simulink library "correlator_library"  (Simulink 6.2)
undefined symbols (not defined in the file or in its folder): BitWidthIn, BramDepth, phase_swtich_counter_width
libraries: xbsIndex_r3 x200, correlator_library x31, fft_library x11
(part 1 of 2)
settings Model: LastModifiedBy=aparsons

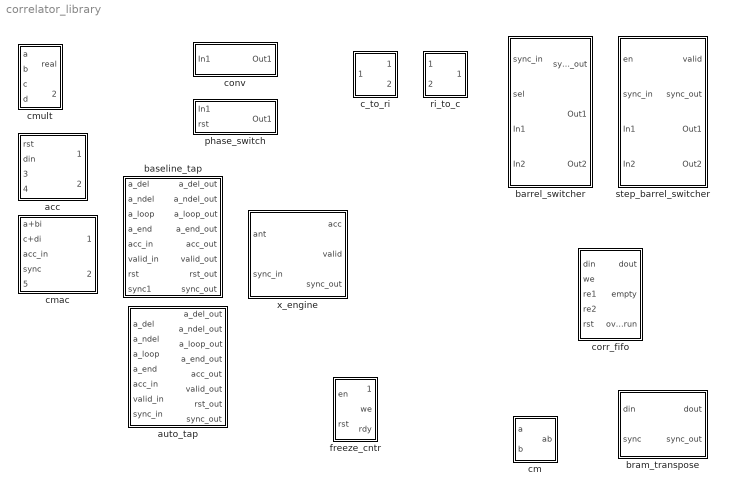
== system correlator_library ==
  acc : Subsystem  mask{BitWidthIn=18, BinPntIn=17, BitWidthOut=18, AccLen=5}
      mask prompts: BitWidthIn "Bit Width In"; BinPntIn "Binary Point In"; BitWidthOut "Bit Width Out"; AccLen "Accumulation Length"
      mask init:
      | BitGrowth = ceil(log2(AccLen));
  auto_tap : Subsystem  mask{AntNum=8, AntSep=1, BitWidthIn=18, BitWidthOut=18, AccLen=32, AddLatency=2, MultLatency=3, use_mult_core=off}
      mask prompts: AntNum "Number of Antennas"; AntSep "Antenna Seperation"; BitWidthIn "Bit Width In"; BitWidthOut "Bit Width Out"; AccLen "Accumulation Length"; AddLatency "Add Latency"; MultLatency "Mult Latency"; use_mult_core "Use Dedicated Multipliers"
      mask init:
      | BitGrowth = ceil(log2(AccLen));
      | AntBits = ceil(log2(AntNum));
      | myname = gcb;
      | set_param(myname, 'LinkStatus', 'inactive');
      | if use_mult_core
      | 	set_param([myname, '/dual_pol_cmac'], 'use_mult_core', 'on');
      | else
      | 	set_param([myname, '/dual_pol_cmac'], 'use_mult_core', 'off');
      | end
  barrel_switcher : Subsystem  mask{n_inputs=1}
      mask prompts: n_inputs "Number of Inputs:"
      mask init:
      | barrel_switcher_mask;
  baseline_tap : Subsystem  mask{AntNum=8, AntSep=1, BitWidthIn=18, BitWidthOut=18, AccLen=32, AddLatency=2, MultLatency=3, use_mult_core=off}
      mask prompts: AntNum "Number of Antennas"; AntSep "Antenna Seperation"; BitWidthIn "Bit Width In"; BitWidthOut "Bit Width Out"; AccLen "Accumulation Length"; AddLatency "Add Latency"; MultLatency "Mult Latency"; use_mult_core "Use Dedicated Multipliers"
      mask init: same as correlator_library/auto_tap
  bram_transpose : Subsystem  mask{Rows=6, Cols=2, StartCol=0}
      mask prompts: Rows "Rows of Matrix (data written in): (2^?)"; Cols "Cols of Matrix (data read out): (2^?)"; StartCol "Starting Read-out Phase (Col Number):"
  c_to_ri : Subsystem  mask{BitWidth=BitWidthIn, BinPnt=0}
      mask prompts: BitWidth "Bit Width:"; BinPnt "Binary Point:"
      mask Display:
      | port_label('input', 1, 'C')
      | port_label('output', 1, 'Re')
      | port_label('output', 2, 'Im')
  cm : Subsystem  mask{mult_latency=3, add_latency=1, use_conj=on, use_mult_core=on, n_bits=18, bin_pt=17, quantization=Round  (unbiased: +/- Inf)}
      mask prompts: mult_latency "Mult latency"; add_latency "Add latency"; use_conj "Conjugate 2nd input"; use_mult_core "Use Dedicated Multiplier"; n_bits "Sample Bitwidth"; bin_pt "Binary Point"
      mask init:
      | if use_mult_core
      | 	set_param([gcb,'/cm'], 'use_mult_core','on');
      | else
      | 	set_param([gcb,'/cm'], 'use_mult_core','off');
      | end
      | 
      | if use_conj
      | 	set_param([gcb,'/cm'],'use_conj', 'on');
      | else
      | 	set_param([gcb,'/cm'],'use_conj', 'off');
      | end
      | 
      | q = 'Round  (unbiased: +/- Inf)';
      | if quantization == 1
      |     q = 'Truncate';
      | end
      | set_param([gcb,'/cm'],'quantization', q);
      mask StyleString: edit,edit,checkbox,checkbox,edit,edit,popup(Truncate|Round  (unbiased: +/- Inf))
  cmac : Subsystem  mask{BitWidthIn=18, BitWidthOut=18, AccLen=32, MultLatency=3, AddLatency=2, use_conj=on, use_mult_core=on}
      mask prompts: BitWidthIn "Bit Width In"; BitWidthOut "Bit Width Out"; AccLen "Accumulation Length"; MultLatency "Mult Latency"; AddLatency "Add Latency"; use_conj "Conjugate 2nd Input"; use_mult_core "Use Dedicated Multipliers"
      mask init:
      | BitGrowth = ceil(log2(AccLen));
      | myname = gcb;
      | if use_conj
      | 	set_param([myname, '/cmult'], 'use_conj', 'on');
      | else
      | 	set_param([myname, '/cmult'], 'use_conj', 'off');
      | end
      | if use_mult_core
      | 	set_param([myname, '/cmult'], 'use_mult_core', 'on');
      | else
      | 	set_param([myname, '/cmult'], 'use_mult_core', 'off');
      | end
  cmult : Subsystem  mask{mult_latency=3, add_latency=1, use_conj=off, use_mult_core=on}
      mask prompts: mult_latency "Mult latency:"; add_latency "Add latency:"; use_conj "Conjugate 2nd input"; use_mult_core "Use Dedicated Multiplier"
      mask init:
      | if use_mult_core
      | 	set_param([gcb,'/ac'], 'use_embedded','on');
      | 	set_param([gcb,'/bd'], 'use_embedded','on');
      | 	set_param([gcb,'/bc'], 'use_embedded','on');
      | 	set_param([gcb,'/ad'], 'use_embedded','on');
      | else
      | 	set_param([gcb,'/ac'], 'use_embedded','off');
      | 	set_param([gcb,'/bd'], 'use_embedded','off');
      | 	set_param([gcb,'/bc'], 'use_embedded','off');
      | 	set_param([gcb,'/ad'], 'use_embedded','off');
      | end
      | 
      | if use_conj
      | 	set_param([gcb,'/real_sum'],'mode', 'Addition');
      | 	set_param([gcb,'/imag_sum'],'mode', 'Subtraction');
      | else
      | 	set_param([gcb,'/real_sum'],'mode', 'Subtraction');
      | 	set_param([gcb,'/imag_sum'],'mode', 'Addition');
      | end
  conv : Subsystem
  corr_fifo : Subsystem  mask{FIFOSize=4, percent_nbits=3}
      mask prompts: FIFOSize "Size of FIFO (2^?)"; percent_nbits "Bit Width of % Full"
      mask init:
      | if FIFOSize >= 10,
      | 	depth = [int2str(2^mod(FIFOSize, 10)), 'K'];
      | else,
      | 	depth = int2str(2^FIFOSize);
      | end
      | set_param([gcb, '/FIFO1'], 'depth', depth);
      | set_param([gcb, '/FIFO1'], 'percent_nbits', num2str(percent_nbits));
  freeze_cntr : Subsystem  mask{CounterBits=BramDepth}
      mask prompts: CounterBits "Counter Length (2^?)"
  phase_switch : Subsystem  mask{counter_width=phase_swtich_counter_width}
      mask prompts: counter_width "Counter Width:"
  ri_to_c : Subsystem  mask{test=0}
      mask prompts: test "Mask Parameter 1:"
      mask Display:
      | port_label('input', 1, 'Re')
      | port_label('input', 2, 'Im')
      | port_label('output', 1, 'C')
  step_barrel_switcher : Subsystem  mask{n_inputs=1, step_dir=Down}
      mask prompts: n_inputs "Number of Inputs: (2^?)"; step_dir "Step Direction"
      mask init:
      | step_barrel_switcher_mask;
      mask StyleString: edit,popup(Up|Down)
  x_engine : Subsystem  mask{AntNum=4, BitWidthIn=18, BitWidthOut=18, AccLen=32, AddLatency=2, MultLatency=3, use_mult_core=off}
      mask prompts: AntNum "Number of Antennas"; BitWidthIn "Bit Width of Samples In"; BitWidthOut "Bit Width of Samples Out"; AccLen "Accumulation Length"; AddLatency "Add Latency"; MultLatency "Mult Latency"; use_mult_core "Use Dedicated Multipliers"
      mask init:
      | myname = gcb;
      | set_param(myname, 'LinkStatus', 'inactive');
      | remove_all_blks(myname);
      | set_param([myname, '/ant'], 'Position', [55, 60, 85, 74]);
      | add_block('xbsIndex_r3/Constant', [myname, '/Constant'], 'Name', 'Constant');
      | set_param([myname, '/Constant'], 'Position', [15, 94, 85, 126]);
      | set_param([myname, '/Constant'], 'const', '0');
      | set_param([myname, '/Constant'], 'n_bits', '8 * BitWidthOut');
      | set_param([myname, '/Constant'], 'explicit_period', 'on');
      | add_block('xbsIndex_r3/Constant', [myname, '/Constant1'], 'Name', 'Constant1');
      | set_param([myname, '/Constant1'], 'Position', [15, 129, 85, 161]);
      | set_param([myname, '/Constant1'], 'const', '0');
      | set_param([myname, '/Constant1'], 'n_bits', '1');
      | set_param([myname, '/Constant1'], 'explicit_period', 'on');
      | set_param([myname, '/sync_in'], 'Position', [55, 185, 85, 199]);
      | x = 140;
      | for i=0:ceil(AntNum / 2)
      | 	if i == 0
      | 		stagename = 'auto_tap';
      | 	else
      | 		stagename = ['baseline_tap', num2str(i)];
      | 	end
      | 	thisblk = [myname, '/', stagename];
      | 	if i == 0
      | 		add_block('correlator_library/auto_tap', thisblk, 'Name', stagename);
      | 	else
      | 		add_block('correlator_library/baseline_tap', thisblk, 'Name', stagename);
      | 	end
      | 	set_param(thisblk, 'Position', [x, 52, x + 95, 168]);
      | 	set_param(thisblk, 'AntNum', 'AntNum');
      | 	set_param(thisblk, 'AntSep', num2str(i));
      | 	set_param(thisblk, 'BitWidthIn', 'BitWidthIn');
      | 	set_param(thisblk, 'BitWidthOut', 'BitWidthOut');
      | 	set_param(thisblk, 'AccLen', 'AccLen');
      | 	set_param(thisblk, 'AddLatency', 'AddLatency');
      | 	set_param(thisblk, 'MultLatency', 'MultLatency');
      | 	if use_mult_core,
      | 		set_param(thisblk, 'use_mult_core', 'on');
      | 	else,
      | 		set_param(thisblk, 'use_mult_core', 'off');
      | 	end
      | 	x = x + 135;
      | end
      | add_block('built-in/Terminator', [myname, '/Terminator'], 'Name', 'Terminator');
      | set_param([myname, '/Terminator'], 'Position', [x, 25, x + 20, 45]);
      | add_block('built-in/Terminator', [myname, '/Terminator1'], 'Name', 'Terminator1');
      | set_param([myname, '/Terminator1'], 'Position', [x, 65, x + 20, 85]);
      | add_block('built-in/Terminator', [myname, '/Terminator2'], 'Name', 'Terminator2');
      | set_param([myname, '/Terminator2'], 'Position', [x, 105, x + 20, 125]);
      | set_param([myname, '/acc'], 'Position', [x, 160, x + 30, 174]);
      | set_param([myname, '/valid'], 'Position', [x, 190, x + 30, 204]);
      | set_param([myname, '/sync_out'], 'Position', [x, 220, x + 30, 234]);
      | 
      | add_line(myname, 'ant/1', 'auto_tap/1', 'autorouting', 'on');
      | add_line(myname, 'ant/1', 'auto_tap/2', 'autorouting', 'on');
      | add_line(myname, 'Constant/1', 'auto_tap/5', 'autorouting', 'on');
      | add_line(myname, 'Constant1/1', 'auto_tap/6', 'autorouting', 'on');
      | add_line(myname, 'sync_in/1', 'auto_tap/7', 'autorouting', 'on');
      | add_line(myname, 'auto_tap/3', 'auto_tap/4', 'autorouting', 'on');
      | for i=1:ceil(AntNum / 2)
      | 	if i == 1
      | 		prevblk = 'auto_tap';
      | 	else
      | 		prevblk = ['baseline_tap', num2str(i-1)];
      | 	end
      | 	thisblk = ['baseline_tap', num2str(i)];
      | 	add_line(myname, [thisblk, '/3'], [prevblk, '/3'], 'autorouting', 'on');
      | 	add_line(myname, [prevblk, '/1'], [thisblk, '/1'], 'autorouting', 'on');
      | 	add_line(myname, [prevblk, '/2'], [thisblk, '/2'], 'autorouting', 'on');
      | 	add_line(myname, [prevblk, '/4'], [thisblk, '/4'], 'autorouting', 'on');
      | 	add_line(myname, [prevblk, '/5'], [thisblk, '/5'], 'autorouting', 'on');
      | 	add_line(myname, [prevblk, '/6'], [thisblk, '/6'], 'autorouting', 'on');
      | 	add_line(myname, [prevblk, '/7'], [thisblk, '/7'], 'autorouting', 'on');
      | 	add_line(myname, [prevblk, '/8'], [thisblk, '/8'], 'autorouting', 'on');
      | end
      | i = ceil(AntNum / 2);
      | thisblk = ['baseline_tap', num2str(i)];
      | add_line(myname, [thisblk, '/1'], [thisblk, '/3'], 'autorouting', 'on');
      | add_line(myname, [thisblk, '/2'], 'Terminator/1', 'autorouting', 'on');
      | add_line(myname, [thisblk, '/4'], 'Terminator1/1', 'autorouting', 'on');
      | add_line(myname, [thisblk, '/5'], 'acc/1', 'autorouting', 'on');
      | add_line(myname, [thisblk, '/6'], 'valid/1', 'autorouting', 'on');
      | add_line(myname, [thisblk, '/7'], 'Terminator2/1', 'autorouting', 'on');
      | add_line(myname, [thisblk, '/8'], 'sync_out/1', 'autorouting', 'on');

== system correlator_library/acc ==
  rst : Inport  Port=1  LatchInput=off
  din : Inport  Port=2  LatchInput=off
  acc_in : Inport  Port=3  LatchInput=off
  valid_in : Inport  Port=4  LatchInput=off
  Accumulator : xbsIndex_r3/Accumulator  n_bits=BitWidthIn + BitGrowth  overflow=Wrap  operation=Add  scale=1  explicit_period=on  period=1  rst=on  hasbypass=on  en=off  dbl_ovrd=off  show_param=off  gen_core=off  use_rpm=on
      settings: xl_area=[0, 0, 0, 0, 0, 0, 0]
  Constant : xbsIndex_r3/Constant  const=1  equ=P=C  arith_type=Unsigned  n_bits=1  bin_pt=0  opselect=C  inp2=PCIN>>17  opr=+  inp1=P  carry=CIN  iostate=0  explicit_period=on  period=1  dbl_ovrd=off
  Convert : xbsIndex_r3/Convert  arith_type="Signed  (2's comp)"  n_bits=BitWidthOut  bin_pt=BitWidthOut - BitGrowth - (BitWidthIn - BinPntIn)  quantization="Round  (unbiased: +/- Inf)"  overflow=Wrap  latency=1  explicit_period=on  period=1  dbl_ovrd=off  show_param=on  inserted_by_tool=off  pipeline=off
      settings: xl_area=[0, 0, 0, 0, 0, 0, 0]
  Convert1 : xbsIndex_r3/Convert  arith_type="Signed  (2's comp)"  n_bits=BitWidthIn + BitGrowth  bin_pt=BinPntIn  quantization="Round  (unbiased: +/- Inf)"  overflow=Wrap  latency=1  explicit_period=off  period=1  dbl_ovrd=off  show_param=on  inserted_by_tool=off  pipeline=off
      settings: xl_area=[0, 0, 0, 0, 0, 0, 0]
  Delay : xbsIndex_r3/Delay  Orientation=up  latency=1  reg_retiming=off  explicit_period=off  period=1  en=off  accept_only_valid=off  init_zero=on  dbl_ovrd=off  show_param=off
      settings: xl_area=[0, 0, 0, 0, 0, 0, 0]
  Delay1 : xbsIndex_r3/Delay  latency=1  reg_retiming=off  explicit_period=off  period=1  en=off  accept_only_valid=off  init_zero=on  dbl_ovrd=off  show_param=off
      settings: xl_area=[0, 0, 0, 0, 0, 0, 0]
  Mux2 : xbsIndex_r3/Mux  inputs=2  precision=Full  arith_type="Signed  (2's comp)"  n_bits=0  bin_pt=0  quantization="Round  (unbiased: +/- Inf)"  overflow=Wrap  latency=2  explicit_period=on  period=1  en=off  dbl_ovrd=off  show_param=off  mux_type=off  use_rpm=off  gen_core=off
      settings: xl_area=[0, 0, 0, 0, 0, 0, 0]
  Mux3 : xbsIndex_r3/Mux  inputs=2  precision=Full  arith_type="Signed  (2's comp)"  n_bits=0  bin_pt=0  quantization=Truncate  overflow=Wrap  latency=2  explicit_period=on  period=1  en=off  dbl_ovrd=off  show_param=off  mux_type=off  use_rpm=off  gen_core=off
      settings: xl_area=[0, 0, 0, 0, 0, 0, 0]
  acc_out : Outport
  valid_out : Outport  Port=2
  wires:
  Accumulator/1 -> Convert/1
  Mux2/1 -> acc_out/1
  acc_in/1 -> Mux2/2
  valid_in/1 -> Mux3/2
  Constant/1 -> Mux3/3
  Mux3/1 -> valid_out/1
  din/1 -> Convert1/1
  rst/1 -> Delay1/1
  Delay/1 -> Mux3/1, Mux2/1
  Convert/1 -> Mux2/3
  Convert1/1 -> Accumulator/1
  Delay1/1 -> Accumulator/2, Delay/1

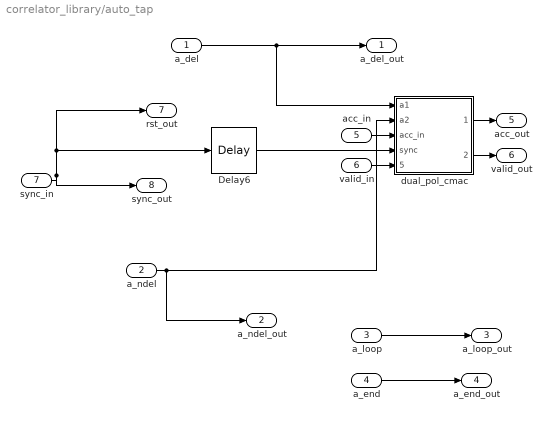
== system correlator_library/auto_tap ==
  a_del : Inport  Port=1  LatchInput=off
  a_ndel : Inport  Port=2  LatchInput=off
  a_loop : Inport  Port=3  LatchInput=off
  a_end : Inport  Port=4  LatchInput=off
  acc_in : Inport  Port=5  LatchInput=off
  valid_in : Inport  Port=6  LatchInput=off
  sync_in : Inport  Port=7  LatchInput=off
  Delay6 : xbsIndex_r3/Delay  latency=1  reg_retiming=off  explicit_period=off  period=1  en=off  accept_only_valid=off  init_zero=on  dbl_ovrd=off  show_param=off
      settings: xl_area=[0, 0, 0, 0, 0, 0, 0]
  dual_pol_cmac : Subsystem  mask{BitWidthIn=BitWidthIn, BitWidthOut=BitWidthOut, AccLen=AccLen, MultLatency=MultLatency, AddLatency=AddLatency, use_mult_core=off}
      mask prompts: BitWidthIn "Bit Width of Sample In"; BitWidthOut "Bit Width of Sample Out"; AccLen "Accumulation Length"; MultLatency "Mult Latency"; AddLatency "Add Latency"; use_mult_core "Use Dedicated Multipliers"
      mask init:
      | myname = gcb;
      | for i=1:4
      | 	if i == 1
      | 		thisblk = '/cmac';
      | 	elseif i == 2
      | 		thisblk = '/cmac1';
      | 	elseif i == 3
      | 		thisblk = '/cmac2';
      | 	elseif i == 4
      | 		thisblk = '/cmac3';
      | 	end
      | 	if use_mult_core
      | 		set_param([myname, thisblk], 'use_mult_core', 'on');
      | 	else
      | 		set_param([myname, thisblk], 'use_mult_core', 'off');
      | 	end
      | end
  a_del_out : Outport
  a_ndel_out : Outport  Port=2
  a_loop_out : Outport  Port=3
  a_end_out : Outport  Port=4
  acc_out : Outport  Port=5
  valid_out : Outport  Port=6
  rst_out : Outport  Port=7
  sync_out : Outport  Port=8
  wires:
  a_loop/1 -> a_loop_out/1
  a_end/1 -> a_end_out/1
  a_ndel/1 -> a_ndel_out/1, dual_pol_cmac/2(a2)
  valid_in/1 -> dual_pol_cmac/5(valid_in)
  dual_pol_cmac/2(valid_out) -> valid_out/1
  acc_in/1 -> dual_pol_cmac/3(acc_in)
  dual_pol_cmac/1(acc_out) -> acc_out/1
  a_del/1 -> a_del_out/1, dual_pol_cmac/1(a1)
  sync_in/1 -> rst_out/1, Delay6/1, sync_out/1
  Delay6/1 -> dual_pol_cmac/4(sync)

== system correlator_library/barrel_switcher ==
  sync_in : Inport  Port=1  LatchInput=off
  sel : Inport  Port=2  LatchInput=off
  In1 : Inport  Port=3  LatchInput=off
  In2 : Inport  Port=4  LatchInput=off
  Delay_sync : xbsIndex_r3/Delay  latency=1  reg_retiming=off  explicit_period=off  period=1  en=off  accept_only_valid=off  init_zero=on  dbl_ovrd=off  show_param=off
      settings: xl_area=[0, 0, 0, 0, 0, 0, 0]
  Mux11 : xbsIndex_r3/Mux  inputs=2  precision=Full  arith_type="Signed  (2's comp)"  n_bits=8  bin_pt=2  quantization=Truncate  overflow=Wrap  latency=1  explicit_period=off  period=1  en=off  dbl_ovrd=off  show_param=off  mux_type=off  use_rpm=off  gen_core=off
      settings: xl_area=[0, 0, 0, 0, 0, 0, 0]
  Mux21 : xbsIndex_r3/Mux  inputs=2  precision=Full  arith_type="Signed  (2's comp)"  n_bits=8  bin_pt=2  quantization=Truncate  overflow=Wrap  latency=1  explicit_period=off  period=1  en=off  dbl_ovrd=off  show_param=off  mux_type=off  use_rpm=off  gen_core=off
      settings: xl_area=[0, 0, 0, 0, 0, 0, 0]
  Slice1 : xbsIndex_r3/Slice  mode=Upper Bit Location + Width  nbits=1  bit1=-0  base1=MSB of Input  bit0=0  base0=LSB of Input  boolean_output=off  explicit_period=off  period=1  dbl_ovrd=off
  sync_out : Outport
  Out1 : Outport  Port=2
  Out2 : Outport  Port=3
  wires:
  sync_in/1 -> Delay_sync/1
  Delay_sync/1 -> sync_out/1
  sel/1 -> Slice1/1
  Slice1/1 -> Mux11/1, Mux21/1
  In1/1 -> Mux11/2, Mux21/3
  Mux11/1 -> Out1/1
  In2/1 -> Mux21/2, Mux11/3
  Mux21/1 -> Out2/1

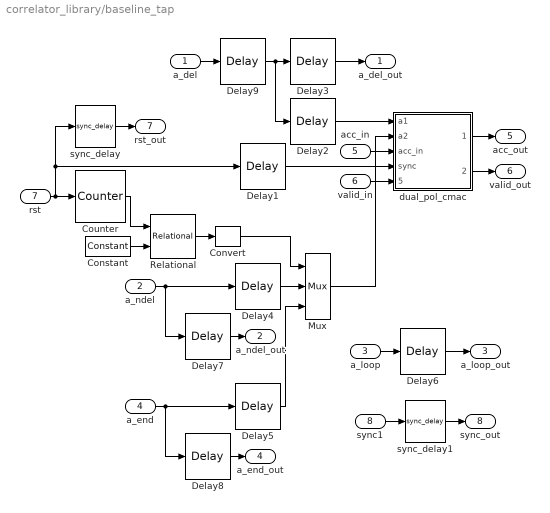
== system correlator_library/baseline_tap ==
  a_del : Inport  Port=1  LatchInput=off
  a_ndel : Inport  Port=2  LatchInput=off
  a_loop : Inport  Port=3  LatchInput=off
  a_end : Inport  Port=4  LatchInput=off
  acc_in : Inport  Port=5  LatchInput=off
  valid_in : Inport  Port=6  LatchInput=off
  rst : Inport  Port=7  LatchInput=off
  sync1 : Inport  Port=8  LatchInput=off
  Constant : xbsIndex_r3/Constant  const=(AntNum - AntSep) * AccLen  equ=P=C  arith_type=Unsigned  n_bits=AntBits + BitGrowth  bin_pt=0  opselect=C  inp2=PCIN>>17  opr=+  inp1=P  carry=CIN  iostate=0  explicit_period=off  period=1  dbl_ovrd=off
  Convert : xbsIndex_r3/Convert  arith_type=Unsigned  n_bits=1  bin_pt=0  quantization=Truncate  overflow=Wrap  latency=0  explicit_period=off  period=1  dbl_ovrd=off  show_param=off  inserted_by_tool=off  pipeline=off
      settings: xl_area=[0, 0, 0, 0, 0, 0, 0]
  Counter : xbsIndex_r3/Counter  cnt_type=Count Limited  n_bits=AntBits + BitGrowth  bin_pt=0  arith_type=Unsigned  start_count=0  cnt_to=AntNum * AccLen - 1  cnt_by_val=1  operation=Up  explicit_period=off  period=1  load_pin=off  rst=on  en=off  dbl_ovrd=off  show_param=off  use_rpm=on  gen_core=off
      settings: xl_area=[0, 0, 0, 0, 0, 0, 0]
  Delay1 : xbsIndex_r3/Delay  latency=2  reg_retiming=off  explicit_period=off  period=1  en=off  accept_only_valid=off  init_zero=on  dbl_ovrd=off  show_param=off
      settings: xl_area=[0, 0, 0, 0, 0, 0, 0]
  Delay2 : xbsIndex_r3/Delay  latency=2  reg_retiming=off  explicit_period=off  period=1  en=off  accept_only_valid=off  init_zero=on  dbl_ovrd=off  show_param=off
      settings: xl_area=[0, 0, 0, 0, 0, 0, 0]
  Delay3 : xbsIndex_r3/Delay  latency=1  reg_retiming=off  explicit_period=off  period=1  en=off  accept_only_valid=off  init_zero=on  dbl_ovrd=off  show_param=off
      settings: xl_area=[0, 0, 0, 0, 0, 0, 0]
  Delay{4..5,7..8} (4 alike) : xbsIndex_r3/Delay  latency=1  reg_retiming=off  explicit_period=on  period=1  en=off  accept_only_valid=off  init_zero=on  dbl_ovrd=off  show_param=off
      settings: xl_area=[0, 0, 0, 0, 0, 0, 0]
  Delay6 : xbsIndex_r3/Delay  latency=2 * AccLen  reg_retiming=off  explicit_period=off  period=1  en=off  accept_only_valid=off  init_zero=on  dbl_ovrd=off  show_param=off
      settings: xl_area=[0, 0, 0, 0, 0, 0, 0]
  Delay9 : xbsIndex_r3/Delay  latency=2 * AccLen  reg_retiming=off  explicit_period=off  period=1  en=off  accept_only_valid=off  init_zero=on  dbl_ovrd=off  show_param=off
      settings: xl_area=[0, 0, 0, 0, 0, 0, 0]
  Mux : xbsIndex_r3/Mux  inputs=2  precision=Full  arith_type="Signed  (2's comp)"  n_bits=8  bin_pt=2  quantization=Truncate  overflow=Wrap  latency=1  explicit_period=off  period=1  en=off  dbl_ovrd=off  show_param=off  mux_type=off  use_rpm=off  gen_core=off
      settings: xl_area=[0, 0, 0, 0, 0, 0, 0]
  Relational : xbsIndex_r3/Relational  mode=a>=b  latency=1  explicit_period=off  period=1  en=off  dbl_ovrd=off  show_param=off
      settings: xl_area=[0, 0, 0, 0, 0, 0, 0]
  dual_pol_cmac : Subsystem  mask{BitWidthIn=BitWidthIn, BitWidthOut=BitWidthOut, AccLen=AccLen, MultLatency=MultLatency, AddLatency=AddLatency, use_mult_core=off}
      mask prompts: BitWidthIn "Bit Width of Sample In"; BitWidthOut "Bit Width of Sample Out"; AccLen "Accumulation Length"; MultLatency "Mult Latency"; AddLatency "Add Latency"; use_mult_core "Use Dedicated Multipliers"
      mask init: same as correlator_library/auto_tap/dual_pol_cmac
  sync_delay : fft_library/sync_delay  DelayLen=AccLen + 1
  sync_delay1 : fft_library/sync_delay  DelayLen=2 * AccLen
  a_del_out : Outport
  a_ndel_out : Outport  Port=2
  a_loop_out : Outport  Port=3
  a_end_out : Outport  Port=4
  acc_out : Outport  Port=5
  valid_out : Outport  Port=6
  rst_out : Outport  Port=7
  sync_out : Outport  Port=8
  wires:
  Delay4/1 -> Mux/2
  Delay5/1 -> Mux/3
  Delay9/1 -> Delay2/1, Delay3/1
  Delay2/1 -> dual_pol_cmac/1(a1)
  Mux/1 -> dual_pol_cmac/2(a2)
  Counter/1 -> Relational/1
  Constant/1 -> Relational/2
  Relational/1 -> Convert/1
  Convert/1 -> Mux/1
  Delay1/1 -> dual_pol_cmac/4(sync)
  rst/1 -> Counter/1, Delay1/1, sync_delay/1
  a_del/1 -> Delay9/1
  dual_pol_cmac/1(acc_out) -> acc_out/1
  acc_in/1 -> dual_pol_cmac/3(acc_in)
  dual_pol_cmac/2(valid_out) -> valid_out/1
  valid_in/1 -> dual_pol_cmac/5(valid_in)
  a_ndel/1 -> Delay4/1, Delay7/1
  a_end/1 -> Delay5/1, Delay8/1
  a_loop/1 -> Delay6/1
  Delay6/1 -> a_loop_out/1
  Delay3/1 -> a_del_out/1
  Delay7/1 -> a_ndel_out/1
  Delay8/1 -> a_end_out/1
  sync_delay/1 -> rst_out/1
  sync_delay1/1 -> sync_out/1
  sync1/1 -> sync_delay1/1

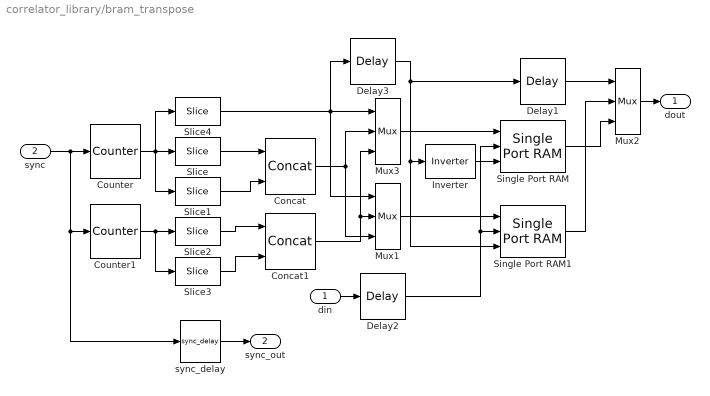
== system correlator_library/bram_transpose ==
  din : Inport  Port=1  LatchInput=off
  sync : Inport  Port=2  LatchInput=off
  Concat : xbsIndex_r3/Concat  num_inputs=2  explicit_period=off  period=1  dbl_ovrd=off
  Concat1 : xbsIndex_r3/Concat  num_inputs=2  explicit_period=off  period=1  dbl_ovrd=off
  Counter : xbsIndex_r3/Counter  cnt_type=Free Running  n_bits=Rows + Cols + 1  bin_pt=0  arith_type=Unsigned  start_count=0  cnt_to=Inf  cnt_by_val=1  operation=Up  explicit_period=on  period=1  load_pin=off  rst=on  en=off  dbl_ovrd=off  show_param=off  use_rpm=on  gen_core=off
      settings: xl_area=[0, 0, 0, 0, 0, 0, 0]
  Counter1 : xbsIndex_r3/Counter  cnt_type=Free Running  n_bits=Rows + Cols + 1  bin_pt=0  arith_type=Unsigned  start_count=StartCol  cnt_to=Inf  cnt_by_val=1  operation=Up  explicit_period=on  period=1  load_pin=off  rst=on  en=off  dbl_ovrd=off  show_param=on  use_rpm=on  gen_core=off
      settings: xl_area=[0, 0, 0, 0, 0, 0, 0]
  Delay1 : xbsIndex_r3/Delay  latency=3  reg_retiming=off  explicit_period=off  period=1  en=off  accept_only_valid=off  init_zero=on  dbl_ovrd=off  show_param=off
      settings: xl_area=[0, 0, 0, 0, 0, 0, 0]
  Delay2 : xbsIndex_r3/Delay  latency=1  reg_retiming=off  explicit_period=off  period=1  en=off  accept_only_valid=off  init_zero=on  dbl_ovrd=off  show_param=off
      settings: xl_area=[0, 0, 0, 0, 0, 0, 0]
  Delay3 : xbsIndex_r3/Delay  latency=1  reg_retiming=off  explicit_period=off  period=1  en=off  accept_only_valid=off  init_zero=on  dbl_ovrd=off  show_param=off
      settings: xl_area=[0, 0, 0, 0, 0, 0, 0]
  Inverter : xbsIndex_r3/Inverter  latency=0  explicit_period=off  period=1  en=off  dbl_ovrd=off  show_param=off
      settings: xl_area=[0, 0, 0, 0, 0, 0, 0]
  Mux1 : xbsIndex_r3/Mux  inputs=2  precision=Full  arith_type="Signed  (2's comp)"  n_bits=8  bin_pt=2  quantization=Truncate  overflow=Wrap  latency=1  explicit_period=off  period=1  en=off  dbl_ovrd=off  show_param=off  mux_type=off  use_rpm=off  gen_core=off
      settings: xl_area=[0, 0, 0, 0, 0, 0, 0]
  Mux2 : xbsIndex_r3/Mux  inputs=2  precision=Full  arith_type="Signed  (2's comp)"  n_bits=8  bin_pt=2  quantization=Truncate  overflow=Wrap  latency=1  explicit_period=off  period=1  en=off  dbl_ovrd=off  show_param=off  mux_type=off  use_rpm=off  gen_core=off
      settings: xl_area=[0, 0, 0, 0, 0, 0, 0]
  Mux3 : xbsIndex_r3/Mux  inputs=2  precision=Full  arith_type="Signed  (2's comp)"  n_bits=8  bin_pt=2  quantization=Truncate  overflow=Wrap  latency=1  explicit_period=off  period=1  en=off  dbl_ovrd=off  show_param=off  mux_type=off  use_rpm=off  gen_core=off
      settings: xl_area=[0, 0, 0, 0, 0, 0, 0]
  Single Port RAM : xbsIndex_r3/Single Port RAM  depth=2^(Rows + Cols)  initVector=0  write_mode=Read Before Write  latency=3  init_zero=on  explicit_period=off  period=1  rst=off  init_reg=0  en=off  dbl_ovrd=off  show_param=off  distributed_mem=off  use_rpm=off  gen_core=off
      settings: xl_area=[0, 0, 0, 0, 0, 0, 0]
  Single Port RAM1 : xbsIndex_r3/Single Port RAM  depth=2^(Rows + Cols)  initVector=0  write_mode=Read Before Write  latency=3  init_zero=on  explicit_period=off  period=1  rst=off  init_reg=0  en=off  dbl_ovrd=off  show_param=off  distributed_mem=off  use_rpm=off  gen_core=off
      settings: xl_area=[0, 0, 0, 0, 0, 0, 0]
  Slice : xbsIndex_r3/Slice  mode=Upper Bit Location + Width  nbits=Cols  bit1=-1  base1=MSB of Input  bit0=0  base0=LSB of Input  boolean_output=off  explicit_period=off  period=1  dbl_ovrd=off
  Slice1 : xbsIndex_r3/Slice  mode=Lower Bit Location + Width  nbits=Rows  bit1=0  base1=MSB of Input  bit0=0  base0=LSB of Input  boolean_output=off  explicit_period=off  period=1  dbl_ovrd=off
  Slice2 : xbsIndex_r3/Slice  mode=Lower Bit Location + Width  nbits=Cols  bit1=-1  base1=MSB of Input  bit0=0  base0=LSB of Input  boolean_output=off  explicit_period=off  period=1  dbl_ovrd=off
  Slice3 : xbsIndex_r3/Slice  mode=Upper Bit Location + Width  nbits=Rows  bit1=-1  base1=MSB of Input  bit0=0  base0=LSB of Input  boolean_output=off  explicit_period=off  period=1  dbl_ovrd=off
  Slice4 : xbsIndex_r3/Slice  mode=Upper Bit Location + Width  nbits=1  bit1=0  base1=MSB of Input  bit0=0  base0=LSB of Input  boolean_output=on  explicit_period=off  period=1  dbl_ovrd=off
  sync_delay : fft_library/sync_delay  DelayLen=2^(Rows + Cols) + 5
  dout : Outport
  sync_out : Outport  Port=2
  wires:
  Slice3/1 -> Concat1/2
  Slice2/1 -> Concat1/1
  Inverter/1 -> Single Port RAM/3
  Mux2/1 -> dout/1
  Delay1/1 -> Mux2/1
  din/1 -> Delay2/1
  Single Port RAM/1 -> Mux2/3
  Single Port RAM1/1 -> Mux2/2
  Mux1/1 -> Single Port RAM1/1
  Mux3/1 -> Single Port RAM/1
  sync/1 -> Counter/1, Counter1/1, sync_delay/1
  Slice1/1 -> Concat/2
  Slice/1 -> Concat/1
  Concat1/1 -> Mux1/2, Mux3/3
  Concat/1 -> Mux1/3, Mux3/2
  Slice4/1 -> Mux1/1, Mux3/1, Delay3/1
  Delay2/1 -> Single Port RAM/2, Single Port RAM1/2
  Delay3/1 -> Single Port RAM1/3, Inverter/1, Delay1/1
  Counter/1 -> Slice/1, Slice4/1, Slice1/1
  Counter1/1 -> Slice2/1, Slice3/1
  sync_delay/1 -> sync_out/1

== system correlator_library/c_to_ri ==
  In1 : Inport  Port=1  LatchInput=off
  Reinterpret : xbsIndex_r3/Reinterpret  force_arith_type=on  arith_type="Signed  (2's comp)"  force_bin_pt=on  bin_pt=BinPnt  force_valid=on
  Reinterpret1 : xbsIndex_r3/Reinterpret  force_arith_type=on  arith_type="Signed  (2's comp)"  force_bin_pt=on  bin_pt=BinPnt  force_valid=on
  Slice : xbsIndex_r3/Slice  mode=Upper Bit Location + Width  nbits=BitWidth  bit1=0  base1=MSB of Input  bit0=0  base0=LSB of Input  boolean_output=off  explicit_period=off  period=1  dbl_ovrd=off
  Slice1 : xbsIndex_r3/Slice  mode=Lower Bit Location + Width  nbits=BitWidth  bit1=0  base1=MSB of Input  bit0=0  base0=LSB of Input  boolean_output=off  explicit_period=off  period=1  dbl_ovrd=off
  Out1 : Outport
  Out2 : Outport  Port=2
  wires:
  In1/1 -> Slice1/1, Slice/1
  Reinterpret1/1 -> Out2/1
  Reinterpret/1 -> Out1/1
  Slice1/1 -> Reinterpret1/1
  Slice/1 -> Reinterpret/1

== system correlator_library/cm ==
  a : Inport  Port=1  LatchInput=off
  b : Inport  Port=2  LatchInput=off
  c_to_ri : correlator_library/c_to_ri  BitWidth=n_bits  BinPnt=bin_pt
  c_to_ri1 : correlator_library/c_to_ri  BitWidth=n_bits  BinPnt=bin_pt
  cm : Subsystem  mask{mult_latency=mult_latency, add_latency=add_latency, use_conj=on, use_mult_core=on, n_bits=n_bits, bin_pt=bin_pt, quantization=Round  (unbiased: +/- Inf)}
      mask prompts: mult_latency "Mult latency:"; add_latency "Add latency:"; use_conj "Conjugate 2nd input"; use_mult_core "Use Dedicated Multiplier"; n_bits "Output Bitwidth"; bin_pt "Output Binary Point"
      mask init:
      | if use_mult_core
      | 	set_param([gcb,'/ac'], 'use_embedded','on');
      | 	set_param([gcb,'/bd'], 'use_embedded','on');
      | 	set_param([gcb,'/bc'], 'use_embedded','on');
      | 	set_param([gcb,'/ad'], 'use_embedded','on');
      | else
      | 	set_param([gcb,'/ac'], 'use_embedded','off');
      | 	set_param([gcb,'/bd'], 'use_embedded','off');
      | 	set_param([gcb,'/bc'], 'use_embedded','off');
      | 	set_param([gcb,'/ad'], 'use_embedded','off');
      | end
      | 
      | if use_conj
      | 	set_param([gcb,'/real_sum'],'mode', 'Addition');
      | 	set_param([gcb,'/imag_sum'],'mode', 'Subtraction');
      | else
      | 	set_param([gcb,'/real_sum'],'mode', 'Subtraction');
      | 	set_param([gcb,'/imag_sum'],'mode', 'Addition');
      | end
      | q = 'Round  (unbiased: +/- Inf)';
      | if quantization == 1
      |     q = 'Truncate';
      | end
      | set_param([gcb,'/real_sum'],'quantization', q);
      | set_param([gcb,'/imag_sum'],'quantization', q);
      mask StyleString: edit,edit,checkbox,checkbox,edit,edit,popup(Truncate|Round  (unbiased: +/- Inf))
  ri_to_c : correlator_library/ri_to_c  test=0
  ab : Outport
  wires:
  c_to_ri/1 -> cm/1(a)
  c_to_ri/2 -> cm/2(b)
  c_to_ri1/1 -> cm/3(c)
  c_to_ri1/2 -> cm/4(d)
  cm/1(real) -> ri_to_c/1
  cm/2(imag) -> ri_to_c/2
  a/1 -> c_to_ri/1
  ri_to_c/1 -> ab/1
  b/1 -> c_to_ri1/1

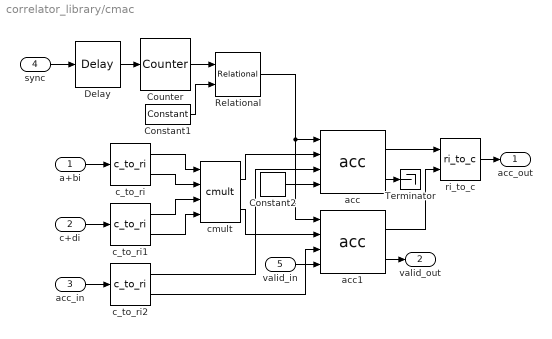
== system correlator_library/cmac ==
  a+bi : Inport  Port=1  LatchInput=off
  c+di : Inport  Port=2  LatchInput=off
  acc_in : Inport  Port=3  LatchInput=off
  sync : Inport  Port=4  LatchInput=off
  valid_in : Inport  Port=5  LatchInput=off
  Constant1 : xbsIndex_r3/Constant  const=0  equ=P=C  arith_type=Unsigned  n_bits=BitGrowth  bin_pt=0  opselect=C  inp2=PCIN>>17  opr=+  inp1=P  carry=CIN  iostate=0  explicit_period=off  period=1  dbl_ovrd=off
  Constant2 : xbsIndex_r3/Constant  const=0  equ=P=C  arith_type=Unsigned  n_bits=1  bin_pt=0  opselect=C  inp2=PCIN>>17  opr=+  inp1=P  carry=CIN  iostate=0  explicit_period=off  period=1  dbl_ovrd=off
  Counter : xbsIndex_r3/Counter  cnt_type=Count Limited  n_bits=BitGrowth  bin_pt=0  arith_type=Unsigned  start_count=0  cnt_to=AccLen - 1  cnt_by_val=1  operation=Up  explicit_period=off  period=1  load_pin=off  rst=on  en=off  dbl_ovrd=off  show_param=off  use_rpm=on  gen_core=off
      settings: xl_area=[0, 0, 0, 0, 0, 0, 0]
  Delay : xbsIndex_r3/Delay  latency=AddLatency + MultLatency - 1  reg_retiming=off  explicit_period=off  period=1  en=off  accept_only_valid=off  init_zero=on  dbl_ovrd=off  show_param=off
      settings: xl_area=[0, 0, 0, 0, 0, 0, 0]
  Relational : xbsIndex_r3/Relational  mode=a=b  latency=1  explicit_period=off  period=1  en=off  dbl_ovrd=off  show_param=off
      settings: xl_area=[0, 0, 0, 0, 0, 0, 0]
  Terminator : Terminator
  acc : correlator_library/acc  BitWidthIn=2*BitWidthIn+1  BinPntIn=2*(BitWidthIn-1)  BitWidthOut=BitWidthOut  AccLen=AccLen
  acc1 : correlator_library/acc  BitWidthIn=2*BitWidthIn+1  BinPntIn=2*(BitWidthIn-1)  BitWidthOut=BitWidthOut  AccLen=AccLen
  c_to_ri : correlator_library/c_to_ri  BitWidth=BitWidthIn  BinPnt=BitWidthIn-1
  c_to_ri1 : correlator_library/c_to_ri  BitWidth=BitWidthIn  BinPnt=BitWidthIn-1
  c_to_ri2 : correlator_library/c_to_ri  BitWidth=BitWidthOut  BinPnt=BitWidthOut - 2 - BitGrowth - 1
  cmult : correlator_library/cmult  mult_latency=MultLatency  add_latency=AddLatency  use_conj=on  use_mult_core=on
  ri_to_c : correlator_library/ri_to_c  test=0
  acc_out : Outport
  valid_out : Outport  Port=2
  wires:
  cmult/1 -> acc/2
  cmult/2 -> acc1/2
  a+bi/1 -> c_to_ri/1
  c_to_ri/1 -> cmult/1
  c_to_ri/2 -> cmult/2
  c+di/1 -> c_to_ri1/1
  c_to_ri1/1 -> cmult/3
  c_to_ri1/2 -> cmult/4
  acc_in/1 -> c_to_ri2/1
  acc/1 -> ri_to_c/1
  acc1/1 -> ri_to_c/2
  ri_to_c/1 -> acc_out/1
  c_to_ri2/1 -> acc/3
  c_to_ri2/2 -> acc1/3
  Relational/1 -> acc/1, acc1/1
  Counter/1 -> Relational/1
  Constant1/1 -> Relational/2
  sync/1 -> Delay/1
  Delay/1 -> Counter/1
  Constant2/1 -> acc/4
  acc/2 -> Terminator/1
  acc1/2 -> valid_out/1
  valid_in/1 -> acc1/4

== system correlator_library/cmult ==
  a : Inport  Port=1  LatchInput=off
  b : Inport  Port=2  LatchInput=off
  c : Inport  Port=3  LatchInput=off
  d : Inport  Port=4  LatchInput=off
  ac : xbsIndex_r3/Mult  precision=Full  arith_type="Signed  (2's comp)"  n_bits=8  bin_pt=2  quantization=Truncate  overflow=Wrap  latency=mult_latency  explicit_period=off  period=1  en=off  dbl_ovrd=off  show_param=off  mult_type=Parallel  oversample=2  use_embedded=on  pipeline=on  use_rpm=on  placement_style=Rectangular Shape  gen_core=off
      settings: xl_area=[0, 0, 0, 0, 0, 0, 0]
  ad : xbsIndex_r3/Mult  precision=Full  arith_type="Signed  (2's comp)"  n_bits=8  bin_pt=2  quantization=Truncate  overflow=Wrap  latency=mult_latency  explicit_period=off  period=1  en=off  dbl_ovrd=off  show_param=off  mult_type=Parallel  oversample=2  use_embedded=on  pipeline=on  use_rpm=on  placement_style=Rectangular Shape  gen_core=off
      settings: xl_area=[0, 0, 0, 0, 0, 0, 0]
  bc : xbsIndex_r3/Mult  precision=Full  arith_type="Signed  (2's comp)"  n_bits=8  bin_pt=2  quantization=Truncate  overflow=Wrap  latency=mult_latency  explicit_period=off  period=1  en=off  dbl_ovrd=off  show_param=off  mult_type=Parallel  oversample=2  use_embedded=on  pipeline=on  use_rpm=on  placement_style=Rectangular Shape  gen_core=off
      settings: xl_area=[0, 0, 0, 0, 0, 0, 0]
  bd : xbsIndex_r3/Mult  precision=Full  arith_type="Signed  (2's comp)"  n_bits=8  bin_pt=2  quantization=Truncate  overflow=Wrap  latency=mult_latency  explicit_period=off  period=1  en=off  dbl_ovrd=off  show_param=off  mult_type=Parallel  oversample=2  use_embedded=on  pipeline=on  use_rpm=on  placement_style=Rectangular Shape  gen_core=off
      settings: xl_area=[0, 0, 0, 0, 0, 0, 0]
  imag_sum : xbsIndex_r3/AddSub  mode=Addition  precision=Full  arith_type=Unsigned  n_bits=8  bin_pt=2  quantization=Truncate  overflow=Wrap  latency=add_latency  explicit_period=off  period=1  use_carryin=off  use_carryout=off  en=off  dbl_ovrd=off  show_param=off  use_core=on  pipeline=off  use_rpm=on  gen_core=off
      settings: xl_area=[0, 0, 0, 0, 0, 0, 0]
  real_sum : xbsIndex_r3/AddSub  mode=Subtraction  precision=Full  arith_type=Unsigned  n_bits=8  bin_pt=2  quantization=Truncate  overflow=Wrap  latency=add_latency  explicit_period=off  period=1  use_carryin=off  use_carryout=off  en=off  dbl_ovrd=off  show_param=off  use_core=on  pipeline=off  use_rpm=on  gen_core=off
      settings: xl_area=[0, 0, 0, 0, 0, 0, 0]
  real : Outport
  imag : Outport  Port=2
  wires:
  ac/1 -> real_sum/1
  bd/1 -> real_sum/2
  bc/1 -> imag_sum/1
  ad/1 -> imag_sum/2
  a/1 -> ad/1, ac/1
  c/1 -> bc/2, ac/2
  b/1 -> bc/1, bd/1
  d/1 -> ad/2, bd/2
  real_sum/1 -> real/1
  imag_sum/1 -> imag/1

== system correlator_library/conv ==
  In1 : Inport  Port=1  LatchInput=off
  Concat : xbsIndex_r3/Concat  num_inputs=2  explicit_period=off  period=1  dbl_ovrd=off
  Inverter : xbsIndex_r3/Inverter  latency=0  explicit_period=off  period=1  en=off  dbl_ovrd=off  show_param=off
      settings: xl_area=[0, 0, 0, 0, 0, 0, 0]
  Reinterpret : xbsIndex_r3/Reinterpret  force_arith_type=on  arith_type="Signed  (2's comp)"  force_bin_pt=on  bin_pt=7  force_valid=on
  Slice : xbsIndex_r3/Slice  mode=Upper Bit Location + Width  nbits=1  bit1=0  base1=MSB of Input  bit0=0  base0=LSB of Input  boolean_output=off  explicit_period=off  period=1  dbl_ovrd=off
  Slice1 : xbsIndex_r3/Slice  mode=Lower Bit Location + Width  nbits=7  bit1=0  base1=MSB of Input  bit0=0  base0=LSB of Input  boolean_output=off  explicit_period=off  period=1  dbl_ovrd=off
  Out1 : Outport
  wires:
  In1/1 -> Slice1/1, Slice/1
  Slice/1 -> Inverter/1
  Inverter/1 -> Concat/1
  Slice1/1 -> Concat/2
  Concat/1 -> Reinterpret/1
  Reinterpret/1 -> Out1/1

== system correlator_library/corr_fifo ==
  din : Inport  Port=1  LatchInput=off
  we : Inport  Port=2  LatchInput=off
  re1 : Inport  Port=3  LatchInput=off
  re2 : Inport  Port=4  LatchInput=off
  rst : Inport  Port=5  LatchInput=off
  FIFO1 : xbsIndex_r3/FIFO  depth=16  percent_nbits=3  store_only_valid=on  init_zero=on  explicit_period=on  period=1  rst=on  en=off  use_almost_empty=off  almost_empty_offset=6  use_almost_full=off  almost_full_offset=6  dbl_ovrd=off  show_param=off  mem_type=Block RAM  gen_core=off
      settings: xl_area=[0, 0, 0, 0, 0, 0, 0]
  Logical : xbsIndex_r3/Logical  Orientation=up  logical_function=OR  inputs=2  precision=Full  arith_type=Unsigned  n_bits=8  bin_pt=2  align_bp=on  latency=0  explicit_period=off  period=1  en=off  dbl_ovrd=off  show_param=off
      settings: xl_area=[0, 0, 0, 0, 0, 0, 0]
  Logical1 : xbsIndex_r3/Logical  logical_function=AND  inputs=2  precision=Full  arith_type=Unsigned  n_bits=8  bin_pt=2  align_bp=on  latency=0  explicit_period=off  period=1  en=off  dbl_ovrd=off  show_param=off
      settings: xl_area=[0, 0, 0, 0, 0, 0, 0]
  Logical2 : xbsIndex_r3/Logical  logical_function=AND  inputs=2  precision=Full  arith_type=Unsigned  n_bits=8  bin_pt=2  align_bp=on  latency=1  explicit_period=off  period=1  en=off  dbl_ovrd=off  show_param=off
      settings: xl_area=[0, 0, 0, 0, 0, 0, 0]
  Terminator : Terminator
  dout : Outport
  empty : Outport  Port=2
  overrun : Outport  Port=3
  wires:
  we/1 -> FIFO1/2, Logical2/2
  FIFO1/1 -> dout/1
  din/1 -> FIFO1/1
  Logical2/1 -> Logical/2, overrun/1
  FIFO1/4 -> Logical2/1
  FIFO1/2 -> empty/1
  Logical/1 -> FIFO1/4
  rst/1 -> Logical/1
  FIFO1/3 -> Terminator/1
  Logical1/1 -> FIFO1/3
  re1/1 -> Logical1/1
  re2/1 -> Logical1/2

== system correlator_library/freeze_cntr ==
  en : Inport  Port=1  LatchInput=off
  rst : Inport  Port=2  LatchInput=off
  Constant5 : xbsIndex_r3/Constant  const=2^CounterBits - 1  equ=P=C  arith_type=Unsigned  n_bits=CounterBits  bin_pt=0  opselect=C  inp2=PCIN>>17  opr=+  inp1=P  carry=CIN  iostate=0  explicit_period=off  period=1  dbl_ovrd=off
  Counter3 : xbsIndex_r3/Counter  cnt_type=Free Running  n_bits=CounterBits  bin_pt=0  arith_type=Unsigned  start_count=0  cnt_to=1023  cnt_by_val=1  operation=Up  explicit_period=on  period=1  load_pin=off  rst=on  en=on  dbl_ovrd=off  show_param=off  use_rpm=on  gen_core=off
      settings: xl_area=[0, 0, 0, 0, 0, 0, 0]
  Delay1 : xbsIndex_r3/Delay  latency=1  reg_retiming=off  explicit_period=off  period=1  en=off  accept_only_valid=off  init_zero=on  dbl_ovrd=off  show_param=off
      settings: xl_area=[0, 0, 0, 0, 0, 0, 0]
  Inverter : xbsIndex_r3/Inverter  latency=0  explicit_period=off  period=1  en=off  dbl_ovrd=off  show_param=off
      settings: xl_area=[0, 0, 0, 0, 0, 0, 0]
  Inverter1 : xbsIndex_r3/Inverter  latency=0  explicit_period=off  period=1  en=off  dbl_ovrd=off  show_param=off
      settings: xl_area=[0, 0, 0, 0, 0, 0, 0]
  Logical1 : xbsIndex_r3/Logical  logical_function=AND  inputs=2  precision=Full  arith_type=Unsigned  n_bits=8  bin_pt=2  align_bp=on  latency=1  explicit_period=off  period=1  en=off  dbl_ovrd=off  show_param=off
      settings: xl_area=[0, 0, 0, 0, 0, 0, 0]
  Logical5 : xbsIndex_r3/Logical  logical_function=AND  inputs=2  precision=Full  arith_type=Unsigned  n_bits=8  bin_pt=2  align_bp=on  latency=0  explicit_period=off  period=1  en=off  dbl_ovrd=off  show_param=off
      settings: xl_area=[0, 0, 0, 0, 0, 0, 0]
  Relational5 : xbsIndex_r3/Relational  mode=a!=b  latency=0  explicit_period=off  period=1  en=off  dbl_ovrd=off  show_param=off
      settings: xl_area=[0, 0, 0, 0, 0, 0, 0]
  addr : Outport
  we : Outport  Port=2
  rdy : Outport  Port=3
  wires:
  rst/1 -> Counter3/1, Inverter/1
  Logical5/1 -> Counter3/2, Logical1/2
  en/1 -> Logical5/1
  Relational5/1 -> Logical5/2, Inverter1/1
  Constant5/1 -> Relational5/2
  Counter3/1 -> Relational5/1, Delay1/1
  Delay1/1 -> addr/1
  Inverter/1 -> Logical1/1
  Logical1/1 -> we/1
  Inverter1/1 -> rdy/1

== system correlator_library/phase_switch ==
  In1 : Inport  Port=1  LatchInput=off
  rst : Inport  Port=2  LatchInput=off
  Counter : xbsIndex_r3/Counter  cnt_type=Count Limited  n_bits=counter_width  bin_pt=0  arith_type=Unsigned  start_count=0  cnt_to=Inf  cnt_by_val=1  operation=Up  explicit_period=off  period=1  load_pin=off  rst=on  en=off  dbl_ovrd=off  show_param=off  use_rpm=on  gen_core=off
      settings: xl_area=[0, 0, 0, 0, 0, 0, 0]
  Delay : xbsIndex_r3/Delay  latency=2  reg_retiming=off  explicit_period=off  period=1  en=off  accept_only_valid=off  init_zero=on  dbl_ovrd=off  show_param=off
      settings: xl_area=[0, 0, 0, 0, 0, 0, 0]
  Mux : xbsIndex_r3/Mux  inputs=2  precision=Full  arith_type="Signed  (2's comp)"  n_bits=8  bin_pt=2  quantization=Truncate  overflow=Wrap  latency=0  explicit_period=off  period=1  en=off  dbl_ovrd=off  show_param=off  mux_type=off  use_rpm=off  gen_core=off
      settings: xl_area=[0, 0, 0, 0, 0, 0, 0]
  Negate : xbsIndex_r3/Negate  precision=Full  arith_type=Unsigned  n_bits=8  bin_pt=2  quantization=Truncate  overflow=Wrap  latency=2  explicit_period=off  period=1  en=off  dbl_ovrd=off  use_core=on  show_param=off  use_rpm=on  gen_core=off
      settings: xl_area=[0, 0, 0, 0, 0, 0, 0]
  Slice : xbsIndex_r3/Slice  mode=Upper Bit Location + Width  nbits=1  bit1=0  base1=MSB of Input  bit0=0  base0=LSB of Input  boolean_output=on  explicit_period=off  period=1  dbl_ovrd=off
  Out1 : Outport
  wires:
  Negate/1 -> Mux/2
  Delay/1 -> Mux/3
  In1/1 -> Negate/1, Delay/1
  Mux/1 -> Out1/1
  Counter/1 -> Slice/1
  rst/1 -> Counter/1
  Slice/1 -> Mux/1

== system correlator_library/ri_to_c ==
  In1 : Inport  Port=1  LatchInput=off
  In2 : Inport  Port=2  LatchInput=off
  Concat : xbsIndex_r3/Concat  num_inputs=2  explicit_period=off  period=1  dbl_ovrd=off
  Reinterpret : xbsIndex_r3/Reinterpret  force_arith_type=on  arith_type=Unsigned  force_bin_pt=on  bin_pt=0  force_valid=on
  Reinterpret1 : xbsIndex_r3/Reinterpret  force_arith_type=on  arith_type=Unsigned  force_bin_pt=on  bin_pt=0  force_valid=on
  Out1 : Outport
  wires:
  Reinterpret/1 -> Concat/1
  Reinterpret1/1 -> Concat/2
  In1/1 -> Reinterpret/1
  Concat/1 -> Out1/1
  In2/1 -> Reinterpret1/1

== system correlator_library/step_barrel_switcher ==
  en : Inport  Port=1  LatchInput=off
  sync_in : Inport  Port=2  LatchInput=off
  In1 : Inport  Port=3  LatchInput=off
  In2 : Inport  Port=4  LatchInput=off
  Counter : xbsIndex_r3/Counter  cnt_type=Free Running  n_bits=n_inputs  bin_pt=0  arith_type=Unsigned  start_count=0  cnt_to=Inf  cnt_by_val=1  operation=Down  explicit_period=off  period=1  load_pin=off  rst=on  en=on  dbl_ovrd=off  show_param=off  use_rpm=on  gen_core=off
      settings: xl_area=[0, 0, 0, 0, 0, 0, 0]
  Delay : xbsIndex_r3/Delay  latency=2  reg_retiming=off  explicit_period=off  period=1  en=off  accept_only_valid=off  init_zero=on  dbl_ovrd=off  show_param=off
      settings: xl_area=[0, 0, 0, 0, 0, 0, 0]
  bs : correlator_library/barrel_switcher  n_inputs=1
  valid : Outport
  sync_out : Outport  Port=2
  Out1 : Outport  Port=3
  Out2 : Outport  Port=4
  wires:
  en/1 -> Delay/1, Counter/2
  Delay/1 -> valid/1
  sync_in/1 -> Counter/1, bs/1
  Counter/1 -> bs/2
  bs/1 -> sync_out/1
  In1/1 -> bs/3
  bs/2 -> Out1/1
  In2/1 -> bs/4
  bs/3 -> Out2/1

== system correlator_library/x_engine ==
  ant : Inport  Port=1  LatchInput=off
  sync_in : Inport  Port=2  LatchInput=off
  Constant : xbsIndex_r3/Constant  const=0  equ=P=C  arith_type=Unsigned  n_bits=8 * BitWidthOut  bin_pt=0  opselect=C  inp2=PCIN>>17  opr=+  inp1=P  carry=CIN  iostate=0  explicit_period=on  period=1  dbl_ovrd=off
  Constant1 : xbsIndex_r3/Constant  const=0  equ=P=C  arith_type=Unsigned  n_bits=1  bin_pt=0  opselect=C  inp2=PCIN>>17  opr=+  inp1=P  carry=CIN  iostate=0  explicit_period=on  period=1  dbl_ovrd=off
  Terminator : Terminator
  Terminator1 : Terminator
  Terminator2 : Terminator
  auto_tap : Subsystem  AncestorBlock=correlator_library/auto_tap  mask{AntNum=AntNum, AntSep=0, BitWidthIn=BitWidthIn, BitWidthOut=BitWidthOut, AccLen=AccLen, AddLatency=AddLatency, MultLatency=MultLatency, use_mult_core=off}
      mask prompts: AntNum "Number of Antennas"; AntSep "Antenna Seperation"; BitWidthIn "Bit Width In"; BitWidthOut "Bit Width Out"; AccLen "Accumulation Length"; AddLatency "Add Latency"; MultLatency "Mult Latency"; use_mult_core "Use Dedicated Multipliers"
      mask init: same as correlator_library/auto_tap
  baseline_tap1 : Subsystem  AncestorBlock=correlator_library/baseline_tap  mask{AntNum=AntNum, AntSep=1, BitWidthIn=BitWidthIn, BitWidthOut=BitWidthOut, AccLen=AccLen, AddLatency=AddLatency, MultLatency=MultLatency, use_mult_core=off}
      mask prompts: AntNum "Number of Antennas"; AntSep "Antenna Seperation"; BitWidthIn "Bit Width In"; BitWidthOut "Bit Width Out"; AccLen "Accumulation Length"; AddLatency "Add Latency"; MultLatency "Mult Latency"; use_mult_core "Use Dedicated Multipliers"
      mask init: same as correlator_library/auto_tap
  baseline_tap2 : Subsystem  AncestorBlock=correlator_library/baseline_tap  mask{AntNum=AntNum, AntSep=2, BitWidthIn=BitWidthIn, BitWidthOut=BitWidthOut, AccLen=AccLen, AddLatency=AddLatency, MultLatency=MultLatency, use_mult_core=off}
      mask prompts: AntNum "Number of Antennas"; AntSep "Antenna Seperation"; BitWidthIn "Bit Width In"; BitWidthOut "Bit Width Out"; AccLen "Accumulation Length"; AddLatency "Add Latency"; MultLatency "Mult Latency"; use_mult_core "Use Dedicated Multipliers"
      mask init: same as correlator_library/auto_tap
  acc : Outport
  valid : Outport  Port=2
  sync_out : Outport  Port=3
  wires:
  ant/1 -> auto_tap/1(a_del), auto_tap/2(a_ndel)
  Constant/1 -> auto_tap/5(acc_in)
  Constant1/1 -> auto_tap/6(valid_in)
  sync_in/1 -> auto_tap/7(sync_in)
  auto_tap/3(a_loop_out) -> auto_tap/4(a_end)
  baseline_tap1/3(a_loop_out) -> auto_tap/3(a_loop)
  auto_tap/1(a_del_out) -> baseline_tap1/1(a_del)
  auto_tap/2(a_ndel_out) -> baseline_tap1/2(a_ndel)
  auto_tap/4(a_end_out) -> baseline_tap1/4(a_end)
  auto_tap/5(acc_out) -> baseline_tap1/5(acc_in)
  auto_tap/6(valid_out) -> baseline_tap1/6(valid_in)
  auto_tap/7(rst_out) -> baseline_tap1/7(rst)
  auto_tap/8(sync_out) -> baseline_tap1/8(sync1)
  baseline_tap2/3(a_loop_out) -> baseline_tap1/3(a_loop)
  baseline_tap1/1(a_del_out) -> baseline_tap2/1(a_del)
  baseline_tap1/2(a_ndel_out) -> baseline_tap2/2(a_ndel)
  baseline_tap1/4(a_end_out) -> baseline_tap2/4(a_end)
  baseline_tap1/5(acc_out) -> baseline_tap2/5(acc_in)
  baseline_tap1/6(valid_out) -> baseline_tap2/6(valid_in)
  baseline_tap1/7(rst_out) -> baseline_tap2/7(rst)
  baseline_tap1/8(sync_out) -> baseline_tap2/8(sync1)
  baseline_tap2/1(a_del_out) -> baseline_tap2/3(a_loop)
  baseline_tap2/2(a_ndel_out) -> Terminator/1
  baseline_tap2/4(a_end_out) -> Terminator1/1
  baseline_tap2/5(acc_out) -> acc/1
  baseline_tap2/6(valid_out) -> valid/1
  baseline_tap2/7(rst_out) -> Terminator2/1
  baseline_tap2/8(sync_out) -> sync_out/1
